simulink model "MinSegShield_Demo_M2V5"  (R2015a)
settings: Solver=FixedStepDiscrete  SolverMode=SingleTasking  StartTime=0.0  StopTime=inf  FixedStep=.03  RelTol=1e-3
libraries: MinSegLibrary_M2V5 x2, RASPlib x2
settings Model: SimulationMode=external  ExtModeTrigDuration=2  Creator=Alec  LastModifiedBy=hurstj
settings OptimizationCC: ExpressionDepthLimit=2147483647  OptimizeModelRefInitCode=on  LifeSpan=1
settings DebuggingCC: UnderspecifiedInitializationDetection=Classic  MergeDetectMultiDrivingBlocksExec=none  StateNameClashWarn=warning
settings HardwareCC: ProdBitPerInt=16  ProdBitPerPointer=8  ProdIntDivRoundTo=Zero  ProdEndianess=LittleEndian  ProdWordSize=8  ProdHWDeviceType=Atmel->AVR
settings RTWCC: SystemTargetFile=realtime.tlc  GenerateMakefile=off  TemplateMakefile=realtime.tmf  Description=Real-Time Toolbox  RTWVerbose=off
settings CodeAppCC: CustomSymbolStrType=$N$R$M  InternalIdentifier=Classic
settings ERTTargetCC: CombineOutputUpdateFcns=off  ExtMode=on  ExtModeTransport=3  ExtModeMexArgs=0 7 115200 30  ERTSrcFileBannerTemplate=realtime_code_template.cgt  ERTHdrFileBannerTemplate=realtime_code_template.cgt  ERTDataSrcFileTemplate=realtime_code_template.cgt  ERTDataHdrFileTemplate=realtime_code_template.cgt  ERTCustomFileTemplate=realtime_file_process.tlc

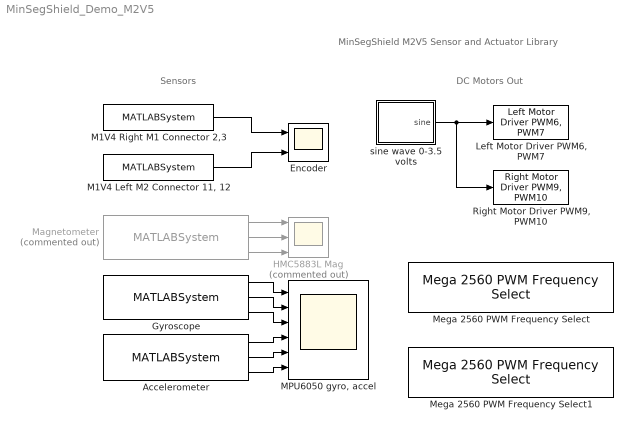
== system MinSegShield_Demo_M2V5 ==
  note: DC Motors Out
  note: Sensors
  note: MinSegShield M2V5 Sensor and Actuator Library
  Accelerometer : MATLABSystem  System=soMPU6050Accel  SimulateUsing=Code generation
      mask Type: soMPU6050Accel
      mask Display:
      | disp('soMPU6050Accel');
      | port_label('output',1,'xaccel');
      | port_label('output',2,'yaccel');
      | port_label('output',3,'zaccel');
  Encoder : Scope  NumInputPorts=2
      settings: TimeRange=10  YMin=-6950~-8950  YMax=-6150~-8425
  Gyroscope : MATLABSystem  System=soMPU6050Gyro  DLPFmode=0
      mask Type: soMPU6050Gyro
      mask Display:
      | disp('soMPU6050Gyro');
      | port_label('output',1,'xvel');
      | port_label('output',2,'yvel');
      | port_label('output',3,'zvel');
  HMC5883L Mag : Scope  Commented=on  NumInputPorts=3
      settings: TimeRange=10  YMin=-5~-210~-267.5  YMax=80~-50~-230  SaveName=ScopeData4
  "Left Motor Driver PWM6, PWM7" : MinSegLibrary_M2V5/Left Motor Driver PWM6, PWM7  Vsupply=5  PWMoffset=0
  "M1V4 Left M2 Connector 11, 12" : MATLABSystem  System=Encoder_arduino  Encoder=4  PinA=11  PinB=12
      mask Type: Encoder_arduino
      mask Display:
      | disp('soEncoder');
      | port_label('output',1,'y');
  M1V4 Right M1 Connector 2,3 : MATLABSystem  System=Encoder_arduino  Encoder=0  PinA=2  PinB=3
      mask Type: Encoder_arduino
      mask Display:
      | disp('soEncoder');
      | port_label('output',1,'y');
  "MPU6050 gyro, accel" : Scope  NumInputPorts=6
      settings: TimeRange=10  YMin=-25000~-40000~-20000~-3000~-1500~3000  YMax=15000~40000~20000~4000~2500~10000
  Magnetometer : MATLABSystem  Commented=on  System=soHMC5883L  SimulateUsing=Code generation
      mask Type: soHMC5883L
      mask Display:
      | disp('soHMC5883L');
      | port_label('output',1,'xmag');
      | port_label('output',2,'ymag');
      | port_label('output',3,'zmag');
  Mega 2560 PWM Frequency Select : RASPlib/Mega 2560 PWM Frequency Select  Frequency=32KHz  Timer=4 - pins 6, 7, 8
  Mega 2560 PWM Frequency Select1 : RASPlib/Mega 2560 PWM Frequency Select  Frequency=32KHz  Timer=2 - pins 9, 10
  "Right Motor Driver PWM9, PWM10 " : MinSegLibrary_M2V5/Right Motor Driver PWM9, PWM10   Vsupply=5  PWMoffset=0
  sine wave 0-3.5 volts : Subsystem
  wires:
  sine wave 0-3.5 volts/1(sine) -> "Right Motor Driver PWM9, PWM10 "/1, "Left Motor Driver PWM6, PWM7"/1
  M1V4 Right M1 Connector 2,3/1 -> Encoder/1
  Gyroscope/1 -> "MPU6050 gyro, accel"/1
  Gyroscope/2 -> "MPU6050 gyro, accel"/2
  Gyroscope/3 -> "MPU6050 gyro, accel"/3
  Accelerometer/1 -> "MPU6050 gyro, accel"/4
  Accelerometer/2 -> "MPU6050 gyro, accel"/5
  Accelerometer/3 -> "MPU6050 gyro, accel"/6
  Magnetometer/1 -> HMC5883L Mag/1
  Magnetometer/2 -> HMC5883L Mag/2
  Magnetometer/3 -> HMC5883L Mag/3
  "M1V4 Left M2 Connector 11, 12"/1 -> Encoder/2

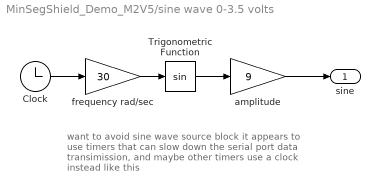
== system MinSegShield_Demo_M2V5/sine wave 0-3.5 volts ==
  note: want to avoid sine wave source block
      | it appears to use timers that can slow down the
      | serial port data transimission, and maybe
      | other timers
      |
      | use a clock instead like this
  Clock : Clock
  Trigonometric Function : Trigonometry
  amplitude : Gain  Gain=9
  frequency rad/sec : Gain  Gain=30
  sine : Outport
  wires:
  Clock/1 -> frequency rad/sec/1
  Trigonometric Function/1 -> amplitude/1
  frequency rad/sec/1 -> Trigonometric Function/1
  amplitude/1 -> sine/1
